simulink model "mass"  (R2020b)
settings: Solver=VariableStepAuto  StartTime=0.0  StopTime=10.0  RelTol=1e-3
settings Model: Creator=99003178  LastModifiedBy=99003178

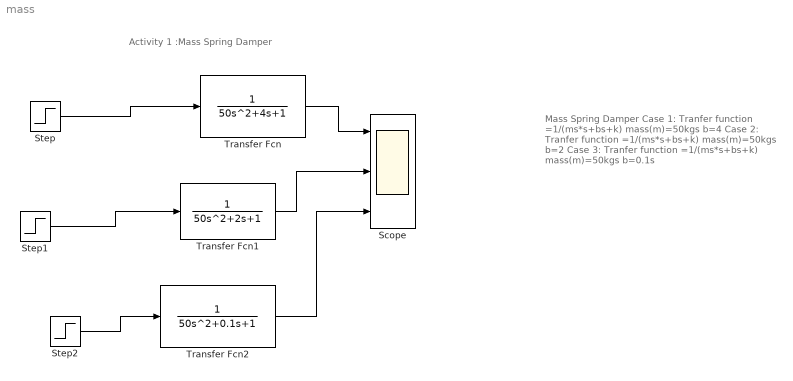
== system mass ==
  note: Mass Spring Damper
      | Case 1:
      | Tranfer function =1/(ms*s+bs+k)
      | mass(m)=50kgs
      | b=4
      | Case 2:
      | Tranfer function =1/(ms*s+bs+k)
      | mass(m)=50kgs
      | b=2
      | Case 3:
      | Tranfer function =1/(ms*s+bs+k)
      | mass(m)=50kgs
      | b=0.1s
  note: Activity 1 :Mass Spring Damper
  Scope : Scope  NumInputPorts=3
  Step : Step  SampleTime=0
  Step1 : Step  SampleTime=0
  Step2 : Step  SampleTime=0
  Transfer Fcn : TransferFcn  Denominator=[50 4 1]
  Transfer Fcn1 : TransferFcn  Denominator=[50 2 1]
  Transfer Fcn2 : TransferFcn  Denominator=[50 0.1 1]
  wires:
  Step/1 -> Transfer Fcn/1
  Transfer Fcn/1 -> Scope/1
  Step1/1 -> Transfer Fcn1/1
  Transfer Fcn1/1 -> Scope/2
  Step2/1 -> Transfer Fcn2/1
  Transfer Fcn2/1 -> Scope/3
